simulink model "Copy_of_LidarModel"  (R2021b)
settings: Solver=VariableStepAuto  StartTime=0.0  StopTime=50  RelTol=1e-3
PreLoadFcn:
  | % Load reference path for recorded drive segment
  | xData   = load('refPosesX.mat');
  | yData   = load('refPosesY.mat');
  | yawData = load('refPosesT.mat');
  | 
  | % Set up workspace variables used by model
  | refPosesX = xData.refPosesX;
  | refPosesY = yData.refPosesY;
  | refPosesT = yawData.refPosesT;
  | 
  | % Load INS measurement
  | insMeasurement = load('insMeasurement.mat');
  | insMeasurement = insMeasurement.insMeasurement;
libraries: sim3dphyssensorlib x1, sim3dlib x1, sim3dautolib x1
settings Model: Creator=The MathWorks, Inc.  LastModifiedBy=Obama
settings SolverCC: AlgebraicLoopSolver=TrustRegion
settings DebuggingCC: SymbolicDimsDataTypeCodeGenerationDiagnostic=none  SFMachineParentedDataDiag=warning

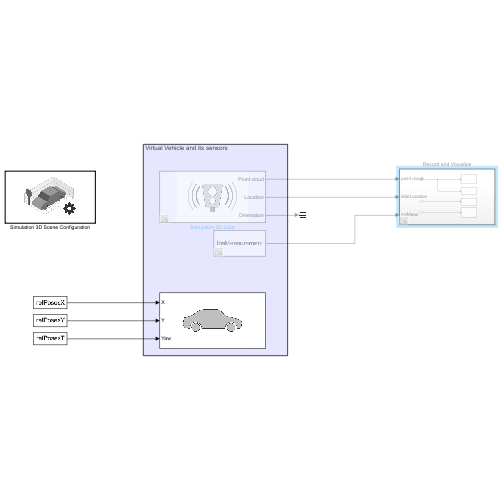
[thumbnail: Simulink's stored preview of the top-level diagram]
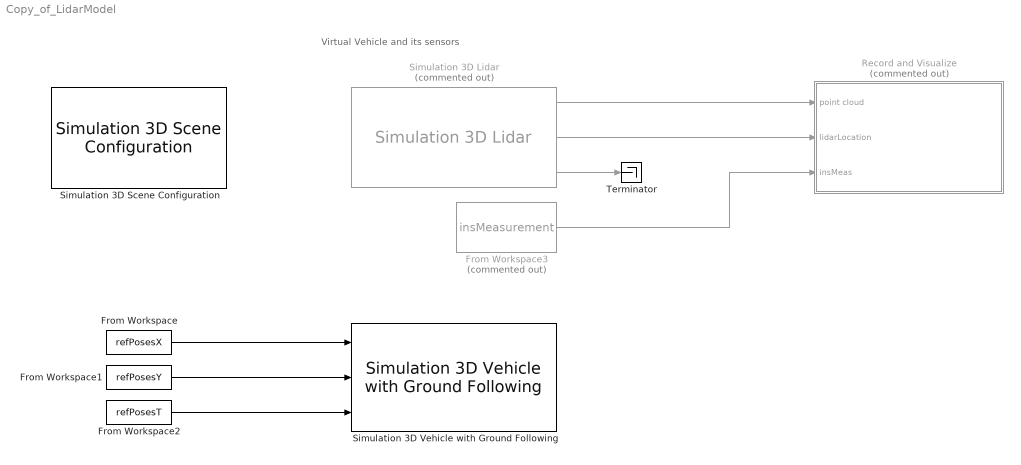
== system Copy_of_LidarModel ==
  note: Virtual Vehicle and its sensors
  From Workspace : FromWorkspace  VariableName=refPosesX  OutputAfterFinalValue=Holding final value
  From Workspace1 : FromWorkspace  VariableName=refPosesY  OutputAfterFinalValue=Holding final value
  From Workspace2 : FromWorkspace  VariableName=refPosesT  Interpolate=off  OutputAfterFinalValue=Holding final value
  From Workspace3 : FromWorkspace  Commented=on  VariableName=insMeasurement  SampleTime=0.1  Interpolate=off  OutputAfterFinalValue=Holding final value
  Record and Visualize : Subsystem  Commented=on  TreatAsAtomicUnit=on
  Simulation 3D Lidar : sim3dphyssensorlib/Simulation 3D Lidar  Commented=on  sensorTag=Sim3dSensor1  sensorId=1  sensorName=Sim3dSensor1  vehTagList={'Scene Origin';'SimulinkVehicle1'}  vehTag=SimulinkVehicle1  mountLoc=Roof center  offsetFlag=off  tmountOffset=[0, 0, 0]  rmountOffset=[0, 0, 0]  DetectionRange=90  RangeResolution=0.002  VerticalFOV=40  VerticalResolution=1.25  HorizontalFOV=360  HorizontalResolution=0.332409972299169  DistanceOutportEnabled=off  TransformOutportEnabled=on  SampleTime=0.1  mountPoint=[-0.25 0 1.57000005245209]  mountOrientation=[0 0 0]  aMode=3  ID=1
      settings: SourceProductBaseCode=AE,DR,UV,VE
  Simulation 3D Scene Configuration : sim3dlib/Simulation 3D Scene Configuration  Priority=0  ProjectFormat_internal=Default Scenes  ProjectFormat=Default Scenes  SceneDesc=Curved road  ProjectName=C:\Program Files\MATLAB\R2021b\toolbox\shared\sim3d_projects\automotive_project\UE4\WindowsNoEditor\VehicleSimulation.exe  ScenePath=/Game/Maps/HwStrght  vehTagList={'Scene Origin';'SimulinkVehicle1'}  vehTag=SimulinkVehicle1  OpVisEn=off  Ts=0.1  EnableWindow=on  EnableWeather=off  SunAltitude=40.0  SunAzimuth=90  clouds=10  wind=1  fog=0  rain=0  sensorTag=MainCamera1  sensorId=1  sensorName=MainCamera1  mountLoc=Origin  offsetFlag=off  tmountOffset=[0, 0, 0]  rmountOffset=[0, 0, 0]  HorizontalResolution=1280  VerticalResolution=720  HorizontalFOV=60  mountPoint=[0 0 0]  mountOrientation=[0 0 0]  aMode=3  ID=1
      settings: SourceProductBaseCode=AE,DR,UV,VE
  Simulation 3D Vehicle with Ground Following : sim3dautolib/Simulation 3D Vehicle with Ground Following  Priority=-1  PassVehMesh=Muscle car  PassVehMesh_Internal=Muscle car  MeshPath=/MathWorksSimulation/Vehicles/Muscle/Meshes/SK_MuscleCar.SK_MuscleCar  TrackWidth=1.9  WheelBase=3  WheelRadius=0.35  VehColor=Yellow  VehColor_Internal=Yellow  InitialPos=[refPosesX(1,2), refPosesY(1,2), 0]  InitialRot=[0, 0, refPosesT(1,2)]  ActorName=SimulinkVehicle1  SampleTime=-1  ActorType=SimulinkVehicle  ID=1  aMode=3  ActorTag=SimulinkVehicle1  CoordinateScheme=ISO  VehLightsControl=off  HeadlightColor=[ 1, 1, 1 ]  HighBeamIntensity=100000  LowBeamIntensity=60000  HighBeamConeAngle=70  LowBeamConeAngle=70  LeftHeadlightOrientation=[ 0, 0 ]  RightHeadlightOrientation=[ 0, 0 ]  BrakelightIntensity=500  ReverselightIntensity=500  SignallightIntensity=500  SignallightPeriod=1  SignalPulseWidth=50  TransformOutportEnabled=off
      settings: SourceProductBaseCode=AE,DR,UV,VE
  Terminator : Terminator
  wires:
  From Workspace2/1 -> Simulation 3D Vehicle with Ground Following/3
  From Workspace1/1 -> Simulation 3D Vehicle with Ground Following/2
  From Workspace/1 -> Simulation 3D Vehicle with Ground Following/1
  Simulation 3D Lidar/1 -> Record and Visualize/1(point cloud)
  From Workspace3/1 -> Record and Visualize/3(insMeas)
  Simulation 3D Lidar/2 -> Record and Visualize/2(lidarLocation)
  Simulation 3D Lidar/3 -> Terminator/1

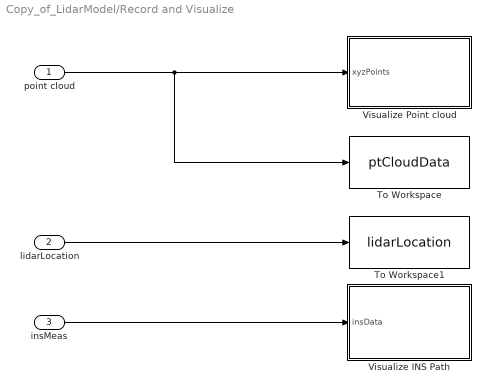
== system Copy_of_LidarModel/Record and Visualize ==
  point cloud : Inport
  lidarLocation : Inport  Port=2
  insMeas : Inport  Port=3
  To Workspace : ToWorkspace  VariableName=ptCloudData  SaveFormat=Structure With Time  SampleTime=-1
  To Workspace1 : ToWorkspace  VariableName=lidarLocation  SaveFormat=Structure With Time  SampleTime=-1
  Visualize INS Path : MATLAB Function  StopFcn=|  TreatAsAtomicUnit=on
      | playerFigure = findall(groot,'type','figure','name','INS Sensor Display');
      | 
      | if ~isempty(playerFigure)
      |     playerFigure = playerFigure(end);
      |     if isvalid(playerFigure)
      |         close(playerFigure);
      |     end
      | end
  Visualize Point cloud : MATLAB Function  StopFcn=|  TreatAsAtomicUnit=on
      | playerFigure = findall(groot,'type','figure','name','Point Cloud Player');
      | 
      | if ~isempty(playerFigure)
      |     playerFigure = playerFigure(end);
      |     if isvalid(playerFigure)
      |         close(playerFigure);
      |     end
      | end
  wires:
  point cloud/1 -> To Workspace/1, Visualize Point cloud/1(xyzPoints)
  insMeas/1 -> Visualize INS Path/1(insData)
  lidarLocation/1 -> To Workspace1/1

== matlab function Copy_of_LidarModel/Record and Visualize/Visualize INS Path ==
  data: insData input
function visualizeINSPath(insData)
%visualizeINSPath Visualize INS path on scene image
%   helperPlotPath plots the path specified by x,y waypoint on the current
%   scene.

% Copyright 2019 The MathWorks, Inc.

coder.extrinsic('helperShowSceneImage', 'figure', 'title', 'movegui', ...
    'isvalid', 'images.roi.Polyline', 'helperUpdatePolyline', 'xlim', 'ylim');

persistent hFig hPoly;

x = insData(1);
y = insData(2);

bufferZone = [30 30];

if isempty(hFig)
    % Query the model to find the scene selection
    sceneName = 'USCityBlock';
    
    % Create a figure and display the scene on it
    hFig = figure('Name', 'INS Sensor Display');
    helperShowSceneImage(sceneName);
    title('INS Sensor Display');
    
    % Move figure to right of screen
    movegui(hFig, 'east')
    
    % Display the path
    hold on
    hPoly = images.roi.Polyline('Parent', gca, 'Position', [x y], 'InteractionsAllowed', 'none');
end

if isvalid(hFig)
    % Update the path with the new point
    helperUpdatePolyline(hPoly, x, y);
    
    xlims = x + bufferZone(1)*[-1 1];
    ylims = y + bufferZone(2)*[-1 1];
    xlim(xlims);
    ylim(ylims);
end
end

== matlab function Copy_of_LidarModel/Record and Visualize/Visualize Point cloud ==
  data: xyzPoints input
function VisualizePointCloud(xyzPoints)
%VisualizePointCloud Display point cloud

coder.extrinsic('isOpen', 'pcplayer')

persistent player;

if isempty(player)
    % Configure axes limits
    xlimits = [-90 90];
    ylimits = [-90 90];
    zlimits = [ -5 40];
    
    % Create a streaming Lidar viewer
    player = pcplayer(xlimits, ylimits, zlimits);
end

if ~isempty(player) && isOpen(player)
    view(player, xyzPoints);
end
